simulink model "sim_all_2019b"  (R2019b)
settings: Solver=VariableStepAuto  StartTime=0.0  StopTime=2000  RelTol=1e-3
values from neighbouring files (symbols this model uses):
  nav_DT = 0.1    [navigation.m]
  nav_giro = 2    [navigation.m]
  nav_h0 = 0    [navigation.m]
  nav_lat0 = cornerC(1)    [navigation.m]
  nav_lon0 = cornerC(2)    [navigation.m]
  nav_plane_AB = coefficient_plane(nav_A,nav_B)    [navigation.m]
  nav_plane_BC = coefficient_plane(nav_B,nav_C)    [navigation.m]
  nav_plane_CD = coefficient_plane(nav_C,nav_D)    [navigation.m]
  nav_plane_DA = coefficient_plane(nav_D,nav_A)    [navigation.m]
undefined symbols (not defined in the file or in its folder): a1, a2, alpha1, alpha2, cornerA, cornerB, cornerC, cornerD, ctrl_clockwise, ctrl_int_bound_or, ctrl_int_bound_pos, ctrl_k_or, ctrl_k_pos, ctrl_Ki_vel, ctrl_Kp_v_pos, ctrl_Kp_vel, ctrl_TAM, ctrl_Ts, ctrl_va_uncontrolled, ctrl_vel_uncontrolled, D, dead_zone_limit, depth, DiscIntNeverNeededParam, distanceFromWall, initInspectedSide, initPoint, mod_A, mod_Cd_F, mod_Cd_M, mod_eta_init, mod_g, mod_h0, mod_Ixx, mod_Iyy, mod_Izz, mod_Kp_dot, mod_lat0, mod_lon0, mod_m, mod_Mq_dot, mod_ni_init, mod_Nr_dot, mod_p1, mod_p2, mod_p3, mod_p4, mod_p5, mod_p6, mod_R, mod_Rm, mod_t1, mod_t2, mod_t3, mod_t4, mod_t5, mod_t6, mod_W, mod_Xu_dot, mod_Yv_dot ... (+44)
libraries: simulink x8, cstblocks x6, simulink_extras x1
(part 1 of 6)
settings Model: PauseTimes=90  Creator=giorg  LastModifiedBy=Marco

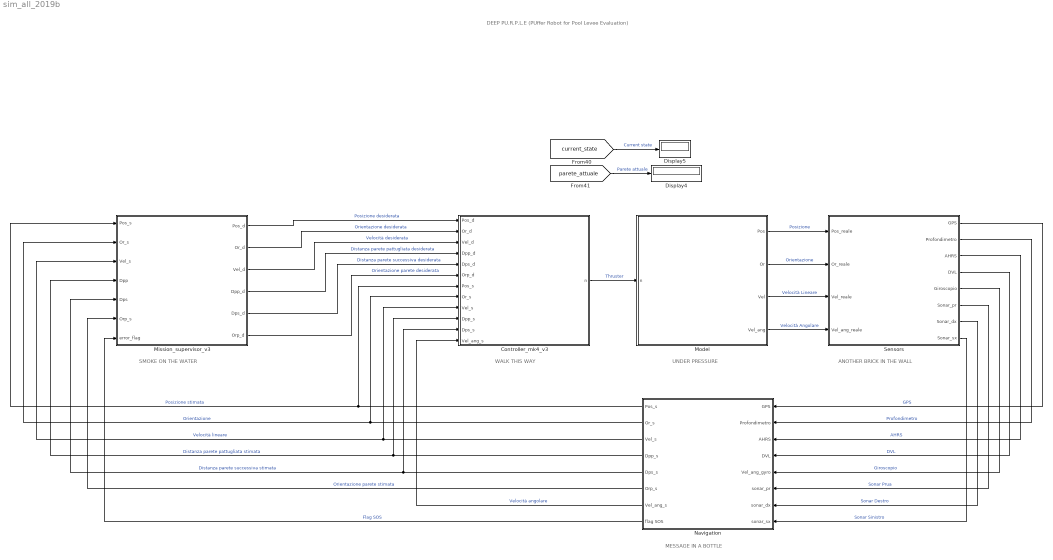
== system sim_all_2019b ==
  note: MESSAGE IN A BOTTLE
  note: ANOTHER BRICK IN THE WALL
  note: UNDER PRESSURE
  note: WALK THIS WAY
  note: SMOKE ON THE WATER
  note: DEEP PU.R.P.L.E
      | (PUffer Robot for Pool Levee Evaluation)
  Controller_mk4_v3 : Subsystem
  Display4 : Display
  Display5 : Display
  Mission_supervisor_v3 : Subsystem
  Model : Subsystem
  Navigation : Subsystem
  Sensors : Subsystem
  wires:
  [parete_attuale] -> Display4/1  "Parete attuale"
  [current_state] -> Display5/1  "Current state"
  Mission_supervisor_v3/1(Pos_d) -> Controller_mk4_v3/1(Pos_d)  "Posizione desiderata"
  Mission_supervisor_v3/2(Or_d) -> Controller_mk4_v3/2(Or_d)  "Orientazione desiderata"
  Mission_supervisor_v3/3(Vel_d) -> Controller_mk4_v3/3(Vel_d)  "Velocità desiderata"
  Mission_supervisor_v3/4(Dpp_d) -> Controller_mk4_v3/4(Dpp_d)  "Distanza parete pattugliata desiderata"
  Mission_supervisor_v3/5(Dps_d) -> Controller_mk4_v3/5(Dps_d)  "Distanza parete successiva desiderata"
  Mission_supervisor_v3/6(Orp_d) -> Controller_mk4_v3/6(Orp_d)  "Orientazione parete desiderata"
  Navigation/1(Pos_s) -> Controller_mk4_v3/7(Pos_s), Mission_supervisor_v3/1(Pos_s)  "Posizione stimata"
  Navigation/2(Or_s) -> Mission_supervisor_v3/2(Or_s), Controller_mk4_v3/8("Or_s ")  "Orientazione"
  Navigation/5(Dps_s) -> Mission_supervisor_v3/5(Dps), Controller_mk4_v3/11(Dps_s)  "Distanza parete successiva stimata"
  Navigation/4(Dpp_s) -> Mission_supervisor_v3/4(Dpp), Controller_mk4_v3/10(Dpp_s)  "Distanza parete pattugliata stimata"
  Navigation/3(Vel_s) -> Mission_supervisor_v3/3(Vel_s), Controller_mk4_v3/9(Vel_s)  "Velocità lineare"
  Controller_mk4_v3/1(n) -> Model/1(n)  "Thruster"
  Model/1(Pos) -> Sensors/1(Pos_reale)  "Posizione"
  Model/2(Or) -> Sensors/2(Or_reale)  "Orientazione"
  Model/4(Vel_ang) -> Sensors/4(Vel_ang_reale)  "Velocità Angolare"
  Navigation/7(Vel_ang_s) -> Controller_mk4_v3/12(Vel_ang_s)  "Velocità angolare"
  Model/3(Vel) -> Sensors/3(Vel_reale)  "Velocità Lineare"
  Sensors/1(GPS) -> Navigation/1(GPS)  "GPS"
  Sensors/5(Giroscopio) -> Navigation/5(Vel_ang_gyro)  "Giroscopio"
  Sensors/2(Profondimetro) -> Navigation/2(Profondimetro)  "Profondimetro"
  Navigation/6(Orp_s) -> Mission_supervisor_v3/6(Orp_s)  "Orientazione parete stimata"
  Navigation/8(flag SOS) -> Mission_supervisor_v3/7(error_flag)  "Flag SOS"
  Sensors/3(AHRS) -> Navigation/3(AHRS)  "AHRS"
  Sensors/6(Sonar_pr) -> Navigation/6(sonar_pr)  "Sonar Prua"
  Sensors/7(Sonar_dx) -> Navigation/7(sonar_dx)  "Sonar Destro"
  Sensors/8(Sonar_sx) -> Navigation/8(sonar_sx)  "Sonar Sinistro"
  Sensors/4(DVL) -> Navigation/4(DVL)  "DVL"

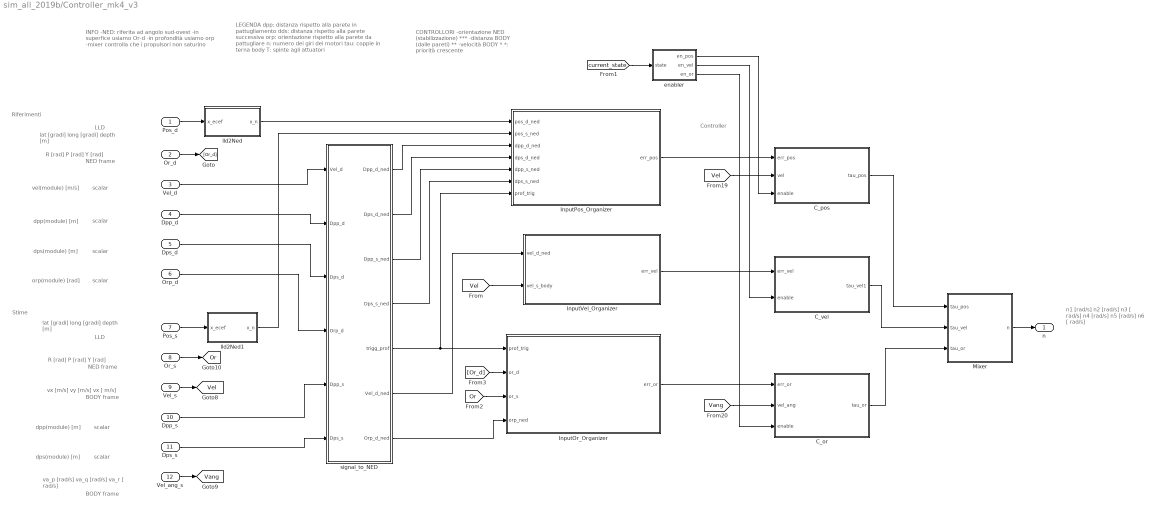
== system sim_all_2019b/Controller_mk4_v3 ==
  note: LEGENDA
      | dpp: distanza rispetto alla parete in pattugliamento
      | dds: distanza rispetto alla parete successiva
      | orp: orientazione rispetto alla parete da pattugliare
      | n: numero dei giri dei motori
      | tau: coppie in terna body
      | T: spinte agli attuatori
  note: CONTROLLORI
      | -orientazione NED (stabilizzazione) ***
      | -distanza BODY (dalle pareti) **
      | -velocità BODY *
      |
      | *: priorità crescente
  note: INFO
      | -NED: riferita ad angolo sud-ovest
      | -in superfice usiamo Or-d
      | -in profondità usiamo orp
      | -mixer controlla che i propulsori non saturino
  note: dpp(module) [m]
  note: LLD
  note: LLD
  note: orp(module) [rad]
  note: scalar
  note: va_p  [rad/s]
      | va_q  [rad/s]
      | va_r [ rad/s]
  note: lat  [gradi]
      | long  [gradi]
      | depth  [m]
  note: NED frame
  note: Controller
  note: dps(module) [m]
  note: BODY frame
  note: R  [rad]
      | P  [rad]
      | Y  [rad]
  note: scalar
  note: scalar
  note: R  [rad]
      | P  [rad]
      | Y  [rad]
  note: Stime
  note: Riferimenti
  note: n1  [rad/s]
      | n2  [rad/s]
      | n3 [ rad/s]
      | n4  [rad/s]
      | n5  [rad/s]
      | n6 [ rad/s]
  note: scalar
  note: vx  [m/s]
      | vy  [m/s]
      | vx [ m/s]
  note: scalar
  note: NED frame
  note: dpp(module) [m]
  note: scalar
  note: dps(module) [m]
  note: vel(module) [m/s]
  note: lat  [gradi]
      | long  [gradi]
      | depth  [m]
  note: BODY frame
  Pos_d : Inport  PortDimensions=[3 1]  SampleTime=ctrl_Ts
  Or_d : Inport  Port=2  PortDimensions=[3 1]  SampleTime=ctrl_Ts
  Vel_d : Inport  Port=3  PortDimensions=[1]  SampleTime=ctrl_Ts
  Dpp_d : Inport  Port=4  PortDimensions=[1]  SampleTime=ctrl_Ts
  Dps_d : Inport  Port=5  PortDimensions=[1]  SampleTime=ctrl_Ts
  Orp_d : Inport  Port=6  PortDimensions=[1]  SampleTime=ctrl_Ts
  Pos_s : Inport  Port=7  PortDimensions=[3 1]  SampleTime=ctrl_Ts
  "Or_s " : Inport  Port=8  PortDimensions=[3 1]  SampleTime=ctrl_Ts
  Vel_s : Inport  Port=9  PortDimensions=[3 1]  SampleTime=ctrl_Ts
  Dpp_s : Inport  Port=10  PortDimensions=[1]  SampleTime=ctrl_Ts
  Dps_s : Inport  Port=11  PortDimensions=[1]  SampleTime=ctrl_Ts
  Vel_ang_s : Inport  Port=12  PortDimensions=[3 1]  SampleTime=ctrl_Ts
  C_or : Subsystem
  C_pos : Subsystem
  C_vel : Subsystem
  InputOr_Organizer : Subsystem
  InputPos_Organizer : Subsystem
  InputVel_Organizer : Subsystem
  Mixer : Subsystem
  enabler : MATLAB Function  TreatAsAtomicUnit=on
  lld2Ned : MATLAB Function  TreatAsAtomicUnit=on
  lld2Ned1 : MATLAB Function  TreatAsAtomicUnit=on
  signal_to_NED : Subsystem
  n : Outport  PortDimensions=[6 1]
  tag scope: Or=global, Vang=global, Vel=global
  wires:
  lld2Ned/1(x_n) -> InputPos_Organizer/1(pos_d_ned)
  InputPos_Organizer/1(err_pos) -> C_pos/1(err_pos)
  enabler/3(en_or) -> C_or/3(enable)
  Pos_s/1 -> lld2Ned1/1(x_ecef)
  [Vel] -> C_pos/2(vel)
  Pos_d/1 -> lld2Ned/1(x_ecef)
  [current_state] -> enabler/1(state)
  [Vang] -> C_or/2(vel_ang)
  C_vel/1(tau_vel1) -> Mixer/2(tau_vel)
  C_or/1(tau_or) -> Mixer/3(tau_or)
  C_pos/1(tau_pos) -> Mixer/1(tau_pos)
  enabler/1(en_pos) -> C_pos/3(enable)
  InputOr_Organizer/1(err_or) -> C_or/1(err_or)
  InputVel_Organizer/1(err_vel) -> C_vel/1(err_vel)
  lld2Ned1/1(x_n) -> InputPos_Organizer/2(pos_s_ned)
  Vel_ang_s/1 -> [Vang]
  signal_to_NED/5(trigg_prof) -> InputPos_Organizer/7(prof_trig), InputOr_Organizer/1(prof_trig)
  signal_to_NED/7(Orp_d_ned) -> InputOr_Organizer/4(orp_ned)
  Vel_d/1 -> signal_to_NED/1(Vel_d)
  Dpp_d/1 -> signal_to_NED/2(Dpp_d)
  Dps_d/1 -> signal_to_NED/3(Dps_d)
  Orp_d/1 -> signal_to_NED/4(Orp_d)
  Dpp_s/1 -> signal_to_NED/5(Dpp_s)
  Dps_s/1 -> signal_to_NED/6(Dps_s)
  signal_to_NED/1(Dpp_d_ned) -> InputPos_Organizer/3(dpp_d_ned)
  signal_to_NED/2(Dps_d_ned) -> InputPos_Organizer/4(dps_d_ned)
  signal_to_NED/3(Dpp_s_ned) -> InputPos_Organizer/5(dpp_s_ned)
  signal_to_NED/4(Dps_s_ned) -> InputPos_Organizer/6(dps_s_ned)
  signal_to_NED/6(Vel_d_ned) -> InputVel_Organizer/1(vel_d_ned)
  "Or_s "/1 -> [Or]
  Vel_s/1 -> [Vel]
  [Vel] -> InputVel_Organizer/2(vel_s_body)
  [Or] -> InputOr_Organizer/3(or_s)
  Or_d/1 -> [Or_d]
  [Or_d] -> InputOr_Organizer/2(or_d)
  enabler/2(en_vel) -> C_vel/2(enable)
  Mixer/1(n) -> n/1

== system sim_all_2019b/Mission_supervisor_v3 ==
  note: Orp [deg]
  note: Vel [m/s]
  note: Dpp [m]
  note: R  [rad]
      | P  [rad]
      | Y  [rad]
  note: ECEF
      | ECEF
      | NED
  note: Roll  [rad]
      | Pitch  [rad]
      | Yaw  [rad]
  note: vx  [m/s]
      | vy  [m/s]
      | vx  [m/s]
  note: BODY frame
  note: ECEF
      | ECEF
      | NED
  note: lat  [gradi]
      | long  [gradi]
      | depth  [m]
  note: Dps [m]
  note: Dpp [m]
  note: Dpp: distanza dalla parete pattugliata
      | Dps: Distanza dalla parete successiva
      | Orp: orientazione rispetto alla parete pattugliata
      | Or_d: orientazione in superficie
  note: Dps [m]
  note: Orp [rad]
  note: lat  [gradi]
      | long  [gradi]
      | depth   [m]
  Pos_s : Inport  PortDimensions=[3 1]
  Or_s : Inport  Port=2  PortDimensions=[3 1]
  Vel_s : Inport  Port=3  PortDimensions=[3 1]
  Dpp : Inport  Port=4  PortDimensions=1
  Dps : Inport  Port=5  PortDimensions=1
  Orp_s : Inport  Port=6  PortDimensions=1
  error_flag : Inport  Port=7  PortDimensions=1
  Display4 : Display
  Display5 : Display
  Mission_Supervisor : Subsystem
  Pos_d : Outport  PortDimensions=[3 1]
  Or_d : Outport  Port=2  PortDimensions=[3 1]
  Vel_d : Outport  Port=3  PortDimensions=1
  Dpp_d : Outport  Port=4  PortDimensions=1
  Dps_d : Outport  Port=5  PortDimensions=1
  Orp_d : Outport  Port=6  PortDimensions=1
  wires:
  [current_state] -> Display5/1
  Mission_Supervisor/5(Dps_d) -> Dps_d/1
  Mission_Supervisor/4(Dpp_d) -> Dpp_d/1
  Dps/1 -> Mission_Supervisor/5(Dps)
  Mission_Supervisor/3(Vel_d) -> Vel_d/1
  error_flag/1 -> Mission_Supervisor/7(error_flag)
  Pos_s/1 -> Mission_Supervisor/1(Pos_S)
  Vel_s/1 -> Mission_Supervisor/3(Vel_S)
  Mission_Supervisor/1(Pos_d) -> Pos_d/1
  Mission_Supervisor/6(Orp_d) -> Orp_d/1
  Dpp/1 -> Mission_Supervisor/4(Dpp)
  [parete_attuale] -> Display4/1
  Orp_s/1 -> Mission_Supervisor/6(Orp_s)
  Mission_Supervisor/2(Or_d) -> Or_d/1
  Or_s/1 -> Mission_Supervisor/2(Or_S)

== system sim_all_2019b/Model ==
  note: Body frame
      | u [m/s]
      | v [m/s]
      | w [m/s]
  note: Body frame
      | p [rad/s]
      | q [rad/s]
      | r [rad/s]
  note: ECEF frame
      | lat [deg]
      | long [deg]
      | depth [m]
  note: NED frame
      | R [rad]
      | P [rad]
      | Y [rad]
  n : Inport  PortDimensions=[6 1]
  Demux : Demux  Outputs=6
  Demux1 : Demux  Outputs=2
  Demux2 : Demux  Outputs=2
  Orientation in Deg : Scope  Commented=on
  Position in ECEF : Scope  Commented=on
  Vehicle Model : Subsystem
  from NED to ECEF : MATLAB Function  TreatAsAtomicUnit=on
  from Rad to Deg : MATLAB Function  TreatAsAtomicUnit=on
  Pos : Outport  PortDimensions=[3 1]
  Or : Outport  Port=2  PortDimensions=[3 1]
  Vel : Outport  Port=3  PortDimensions=[3 1]
  Vel_ang : Outport  Port=4  PortDimensions=[3 1]
  wires:
  n/1 -> Demux/1
  from Rad to Deg/1(eta2_deg) -> Orientation in Deg/1  "eta2_deg"
  Vehicle Model/2(ni) -> Demux1/1
  Demux/3 -> Vehicle Model/3(In3)
  Demux/4 -> Vehicle Model/4(In4)
  from NED to ECEF/1(eta1_ECEF) -> Position in ECEF/1, Pos/1  "eta1_ECEF"
  Vehicle Model/1(eta) -> Demux2/1
  Demux/6 -> Vehicle Model/6(In6)
  Demux/1 -> Vehicle Model/1(In1)
  Demux/5 -> Vehicle Model/5(In5)
  Demux2/1 -> from NED to ECEF/1(eta1)  "Posizione Reale NED"
  Demux1/2 -> Vel_ang/1  "ni2"
  Demux1/1 -> Vel/1  "ni1"
  Demux2/2 -> Or/1, from Rad to Deg/1(eta2)  "eta2"
  Demux/2 -> Vehicle Model/2(In2)

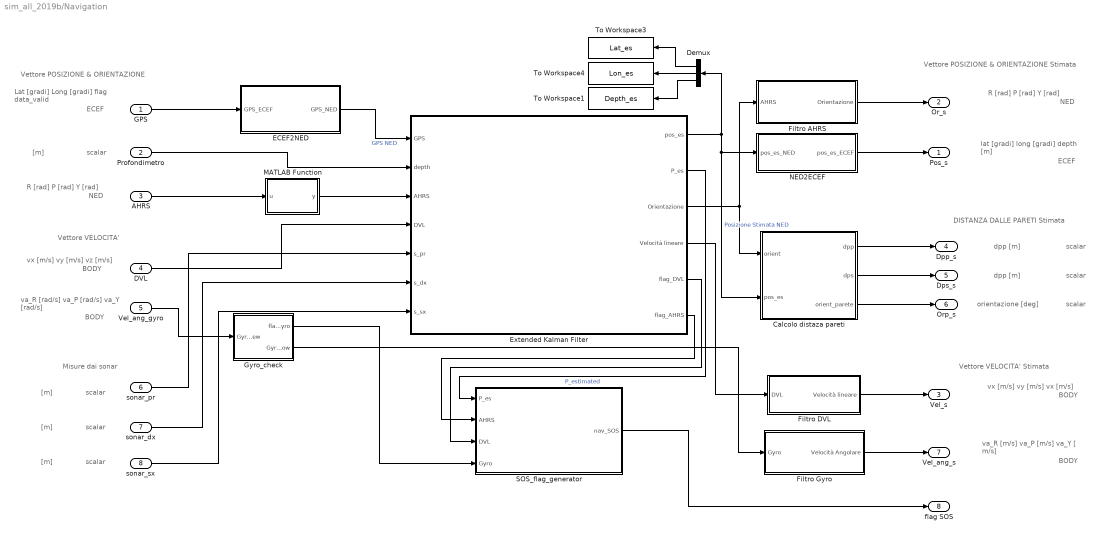
== system sim_all_2019b/Navigation ==
  note: Vettore POSIZIONE & ORIENTAZIONE
  note: vx  [m/s]
      | vy  [m/s]
      | vx  [m/s]
  note: R [rad]
      | P [rad]
      | Y [rad]
  note: vx  [m/s]
      | vy  [m/s]
      | vz  [m/s]
  note: scalar
  note: dpp [m]
  note: [m]
  note: [m]
  note: NED
  note: ECEF
  note: lat  [gradi]
      | long  [gradi]
      | depth   [m]
  note: va_R [rad/s]
      | va_P [rad/s]
      | va_Y [rad/s]
  note: NED
  note: va_R  [m/s]
      | va_P  [m/s]
      | va_Y [ m/s]
  note: BODY
  note: [m]
  note: BODY
  note: Lat  [gradi]
      | Long  [gradi]
      | flag data_valid
  note: ECEF
  note: R  [rad]
      | P  [rad]
      | Y  [rad]
  note: scalar
  note: BODY
  note: scalar
  note: scalar
  note: scalar
  note: scalar
  note: BODY
  note: [m]
  note: Vettore POSIZIONE & ORIENTAZIONE Stimata
  note: Vettore VELOCITA'
  note: DISTANZA DALLE PARETI Stimata
  note: Vettore VELOCITA' Stimata
  note: Misure dai sonar
  note: dpp [m]
  note: orientazione [deg]
  note: scalar
  GPS : Inport  PortDimensions=[3 1]
  Profondimetro : Inport  Port=2  PortDimensions=1
  AHRS : Inport  Port=3  PortDimensions=[3 1]
  DVL : Inport  Port=4  PortDimensions=[3 1]
  Vel_ang_gyro : Inport  Port=5  PortDimensions=[3 1]
  sonar_pr : Inport  Port=6  PortDimensions=1
  sonar_dx : Inport  Port=7  PortDimensions=1
  sonar_sx : Inport  Port=8  PortDimensions=1
  Calcolo distaza pareti : Subsystem
  Demux : Demux  Outputs=3
  ECEF2NED : MATLAB Function  TreatAsAtomicUnit=on
  Extended Kalman Filter : Subsystem  TreatAsAtomicUnit=on
  Filtro AHRS : Subsystem
  Filtro DVL : Subsystem
  Filtro Gyro : Subsystem
  Gyro_check : Subsystem
  MATLAB Function : MATLAB Function  TreatAsAtomicUnit=on
  NED2ECEF : MATLAB Function  TreatAsAtomicUnit=on
  SOS_flag_generator : Subsystem
  To Workspace1 : ToWorkspace  VariableName=Depth_es  SaveFormat=Timeseries  SampleTime=-1
      settings: Decimation=10
  To Workspace3 : ToWorkspace  VariableName=Lat_es  SaveFormat=Timeseries  SampleTime=-1
      settings: Decimation=10
  To Workspace4 : ToWorkspace  VariableName=Lon_es  SaveFormat=Timeseries  SampleTime=-1
      settings: Decimation=10
  Pos_s : Outport  PortDimensions=[3 1]
  Or_s : Outport  Port=2  PortDimensions=[3 1]
  Vel_s : Outport  Port=3  PortDimensions=[3 1]
  Dpp_s : Outport  Port=4  PortDimensions=1
  Dps_s : Outport  Port=5  PortDimensions=1
  Orp_s : Outport  Port=6  PortDimensions=1
  Vel_ang_s : Outport  Port=7  PortDimensions=[3 1]
  flag SOS : Outport  Port=8  PortDimensions=1
  wires:
  Profondimetro/1 -> Extended Kalman Filter/2(depth)
  sonar_pr/1 -> Extended Kalman Filter/5(s_pr)
  sonar_dx/1 -> Extended Kalman Filter/6(s_dx)
  sonar_sx/1 -> Extended Kalman Filter/7(s_sx)
  Extended Kalman Filter/1(pos_es) -> Calcolo distaza pareti/2(pos_es), NED2ECEF/1(pos_es_NED), Demux/1  "Posizione Stimata NED"
  Calcolo distaza pareti/1(dpp) -> Dpp_s/1
  Calcolo distaza pareti/2(dps) -> Dps_s/1
  NED2ECEF/1(pos_es_ECEF) -> Pos_s/1
  GPS/1 -> ECEF2NED/1(GPS_ECEF)
  ECEF2NED/1(GPS_NED) -> Extended Kalman Filter/1(GPS)  "GPS NED"
  Calcolo distaza pareti/3(orient_parete) -> Orp_s/1
  Extended Kalman Filter/2(P_es) -> SOS_flag_generator/1(P_es)  "P_estimated"
  AHRS/1 -> MATLAB Function/1(u)
  Filtro DVL/1(Velocità lineare) -> Vel_s/1
  Filtro AHRS/1(Orientazione) -> Or_s/1
  Filtro Gyro/1(Velocità Angolare) -> Vel_ang_s/1
  MATLAB Function/1(y) -> Extended Kalman Filter/3(AHRS)
  Extended Kalman Filter/3(Orientazione) -> Calcolo distaza pareti/1(orient), Filtro AHRS/1(AHRS)
  Vel_ang_gyro/1 -> Gyro_check/1(Gyro_new)
  Gyro_check/2(Gyro_now) -> Filtro Gyro/1(Gyro)
  Extended Kalman Filter/5(flag_DVL) -> SOS_flag_generator/3(DVL)
  Extended Kalman Filter/6(flag_AHRS) -> SOS_flag_generator/2(AHRS)
  Gyro_check/1(flag_Gyro) -> SOS_flag_generator/4(Gyro)
  SOS_flag_generator/1(nav_SOS) -> flag SOS/1
  DVL/1 -> Extended Kalman Filter/4(DVL)
  Extended Kalman Filter/4(Velocità lineare) -> Filtro DVL/1(DVL)
  Demux/2 -> To Workspace4/1
  Demux/1 -> To Workspace3/1
  Demux/3 -> To Workspace1/1

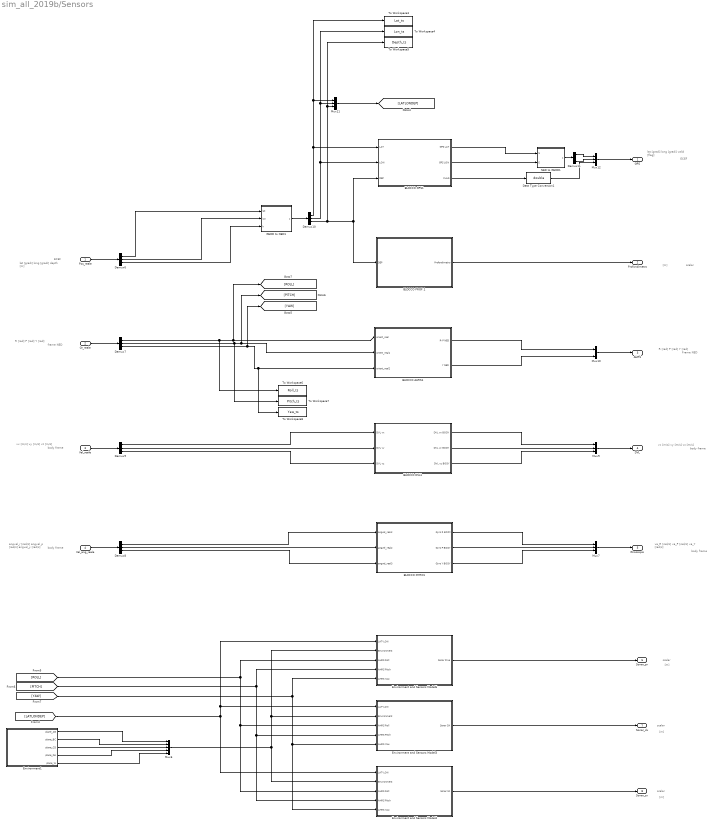
== system sim_all_2019b/Sensors ==
  note: body frame
  note: body frame
  note: ECEF
  note: scalar
  note: [m]
  note: [m]
  note: R  [rad]
      | P  [rad]
      | Y  [rad]
  note: ECEF
  note: va_R [rad/s]
      | va_P [rad/s]
      | va_Y [rad/s]
  note: Frame NED
  note: lat  [gradi]
      | long  [gradi]
      | valid [flag]
  note: body frame
  note: [m]
  note: angvel_r  [rad/s]
      | angvel_p  [rad/s]
      | angvel_y  [rad/s]
  note: vx  [m/s]
      | vy  [m/s]
      | vz  [m/s]
  note: frame NED
  note: lat  [gradi]
      | long  [gradi]
      | depth  [m]
  note: scalar
  note: vx  [m/s]
      | vy  [m/s]
      | vz  [m/s]
  note: scalar
  note: body frame
  note: [m]
  note: scalar
  note: R  [rad]
      | P  [rad]
      | Y  [rad]
  Pos_reale : Inport  PortDimensions=[3 1]
  Or_reale : Inport  Port=2  PortDimensions=[3 1]
  Vel_reale : Inport  Port=3  PortDimensions=[3 1]
  Vel_ang_reale : Inport  Port=4  PortDimensions=[3 1]
  BLOCCO AHRS1 : Subsystem
  BLOCCO DVL1 : Subsystem
  BLOCCO GPS1 : Subsystem
  BLOCCO GYRO1 : Subsystem
  BLOCCO PROF.1 : Subsystem
  Data Type Conversion1 : DataTypeConversion  OutDataTypeStr=double
  Demux{6..10} (5 alike) : Demux  Outputs=3
  Demux11 : Demux  Outputs=2
  Environment and Sensors Model3 : Subsystem
  Environment and Sensors Model4 : Subsystem
  Environment and Sensors Model6 : Subsystem
  Environment1 : MATLAB Function  TreatAsAtomicUnit=on
  GEOD to NED1 : MATLAB Function  TreatAsAtomicUnit=on
  Mux10 : Mux  Inputs=2
  Mux{7,9,11..12} (4 alike) : Mux  Inputs=3
  Mux6 : Mux  Inputs=5
  NED to GEOD1 : MATLAB Function  TreatAsAtomicUnit=on
  To Workspace3 : ToWorkspace  VariableName=Lat_ts  SaveFormat=Timeseries  SampleTime=-1
      settings: Decimation=10
  To Workspace4 : ToWorkspace  VariableName=Lon_ts  SaveFormat=Timeseries  SampleTime=-1
      settings: Decimation=10
  To Workspace5 : ToWorkspace  VariableName=Depth_ts  SaveFormat=Timeseries  SampleTime=-1
      settings: Decimation=10
  To Workspace6 : ToWorkspace  VariableName=Roll_ts  SaveFormat=Timeseries  SampleTime=-1
      settings: Decimation=10
  To Workspace7 : ToWorkspace  VariableName=Pitch_ts  SaveFormat=Timeseries  SampleTime=-1
      settings: Decimation=10
  To Workspace8 : ToWorkspace  VariableName=Yaw_ts  SaveFormat=Timeseries  SampleTime=-1
      settings: Decimation=10
  GPS : Outport  PortDimensions=[3 1]
  Profondimetro : Outport  Port=2  PortDimensions=1
  AHRS : Outport  Port=3  PortDimensions=[3 1]
  DVL : Outport  Port=4  PortDimensions=[3 1]
  Giroscopio : Outport  Port=5  PortDimensions=[3 1]
  Sonar_pr : Outport  Port=6  PortDimensions=1
  Sonar_dx : Outport  Port=7  PortDimensions=1
  Sonar_sx : Outport  Port=8  PortDimensions=1
  wires:
  Environment1/5(plane_W) -> Mux6/5
  Demux10/2 -> BLOCCO GPS1/2("LON "), To Workspace4/1, Mux11/2
  Demux10/1 -> To Workspace3/1, Mux11/1, BLOCCO GPS1/1("LAT ")
  BLOCCO DVL1/2(DVL vy BODY) -> Mux9/2
  Environment and Sensors Model6/1(Sonar Prua) -> Sonar_pr/1
  BLOCCO AHRS1/1(R-P NED) -> Mux10/1
  BLOCCO GYRO1/3(Gyro Y BODY) -> Mux7/3
  Demux9/3 -> BLOCCO DVL1/3(DVL vz)
  Demux10/3 -> BLOCCO GPS1/3(DEP), BLOCCO PROF.1/1(DEP), To Workspace5/1, Mux11/3
  Demux9/2 -> BLOCCO DVL1/2(DVL vy)
  BLOCCO GYRO1/1(Gyro R BODY) -> Mux7/1
  BLOCCO DVL1/1(DVL vx BODY) -> Mux9/1
  BLOCCO AHRS1/2(Y NED) -> Mux10/2
  Environment1/2(plane_BC) -> Mux6/2
  Pos_reale/1 -> Demux6/1
  BLOCCO GYRO1/2(Gyro P BODY) -> Mux7/2
  Vel_ang_reale/1 -> Demux8/1
  Environment1/3(plane_CD) -> Mux6/3
  [YAW] -> Environment and Sensors Model3/5(AHRS Yaw), Environment and Sensors Model4/5(AHRS Yaw), Environment and Sensors Model6/5(AHRS Yaw)
  Mux6/1 -> Environment and Sensors Model3/2(Environment), Environment and Sensors Model6/2(Environment), Environment and Sensors Model4/2(Environment)
  Vel_reale/1 -> Demux9/1
  Demux6/2 -> GEOD to NED1/2(lon)
  Data Type Conversion1/1 -> Mux12/3
  Demux11/2 -> Mux12/2
  Or_reale/1 -> Demux7/1
  Demux8/3 -> BLOCCO GYRO1/3(angvel_real3)
  BLOCCO DVL1/3(DVL vz BODY) -> Mux9/3
  Mux10/1 -> AHRS/1
  Demux7/1 -> To Workspace6/1, BLOCCO AHRS1/1(orient_real), [ROLL]
  Demux7/2 -> To Workspace7/1, BLOCCO AHRS1/2(orient_real1), [PITCH]
  Demux6/1 -> GEOD to NED1/1(lat)
  [PITCH] -> Environment and Sensors Model6/4(AHRS Pitch), Environment and Sensors Model3/4(AHRS Pitch), Environment and Sensors Model4/4(AHRS Pitch)
  Demux8/1 -> BLOCCO GYRO1/1(angvel_rea1l)
  Demux7/3 -> To Workspace8/1, BLOCCO AHRS1/3(orient_real2), [YAW]
  Demux6/3 -> GEOD to NED1/3(h)
  Mux11/1 -> [LATLONDEP]
  Mux9/1 -> DVL/1
  Environment and Sensors Model4/1(Sonar SX) -> Sonar_sx/1
  Mux7/1 -> Giroscopio/1
  BLOCCO GPS1/3(FLAG) -> Data Type Conversion1/1
  BLOCCO PROF.1/1(Profondimetro) -> Profondimetro/1
  [ROLL] -> Environment and Sensors Model6/3(AHRS Roll), Environment and Sensors Model3/3(AHRS Roll), Environment and Sensors Model4/3(AHRS Roll)
  BLOCCO GPS1/2("GPS LON ") -> NED to GEOD1/2(E)
  GEOD to NED1/1(z) -> Demux10/1
  Demux8/2 -> BLOCCO GYRO1/2(angvel_real2)
  Demux9/1 -> BLOCCO DVL1/1("DVL vx ")
  BLOCCO GPS1/1("GPS LAT ") -> NED to GEOD1/1(N)
  [LATLONDEP] -> Environment and Sensors Model3/1(LAT-LON), Environment and Sensors Model6/1(LAT-LON), Environment and Sensors Model4/1(LAT-LON)
  NED to GEOD1/1(z) -> Demux11/1
  Demux11/1 -> Mux12/1
  Environment1/1(plane_AB) -> Mux6/1
  Environment and Sensors Model3/1(Sonar DX) -> Sonar_dx/1
  Environment1/4(plane_DA) -> Mux6/4
  Mux12/1 -> GPS/1

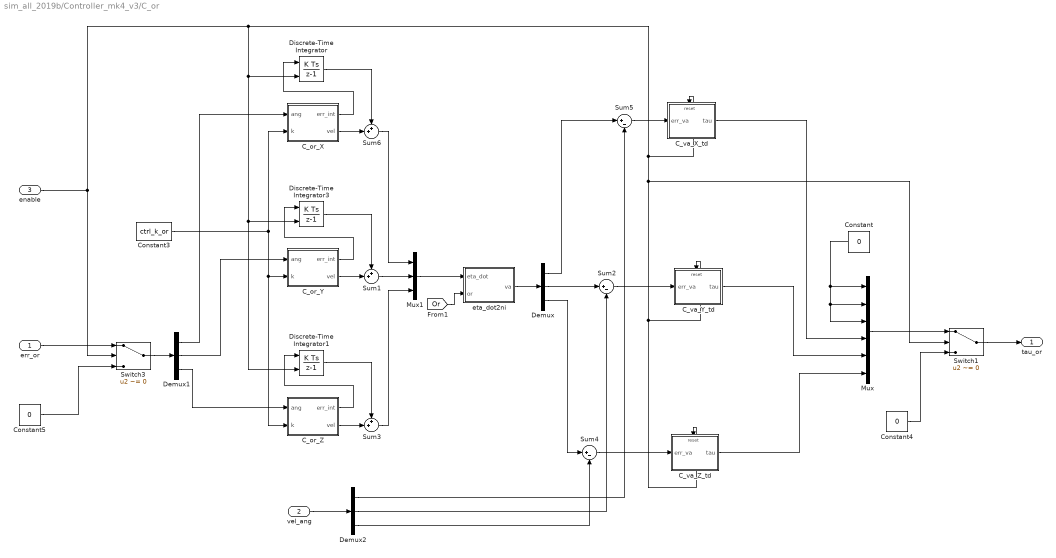
== system sim_all_2019b/Controller_mk4_v3/C_or ==
  err_or : Inport
  vel_ang : Inport  Port=2
  enable : Inport  Port=3
  C_or_X : MATLAB Function  TreatAsAtomicUnit=on  SystemSampleTime=ctrl_Ts
  C_or_Y : MATLAB Function  TreatAsAtomicUnit=on  SystemSampleTime=ctrl_Ts
  C_or_Z : MATLAB Function  TreatAsAtomicUnit=on  SystemSampleTime=ctrl_Ts
  C_va_X_td : Subsystem  TreatAsAtomicUnit=on
  C_va_Y_td : Subsystem  TreatAsAtomicUnit=on
  C_va_Z_td : Subsystem  TreatAsAtomicUnit=on
  Constant : Constant  Value=0
  Constant3 : Constant  Value=ctrl_k_or
  Constant4 : Constant  Value=0
  Constant5 : Constant  Value=0
  Demux : Demux  Outputs=3
  Demux1 : Demux  Outputs=3
  Demux2 : Demux  Outputs=3
  Discrete-Time Integrator : DiscreteIntegrator  gainval=ctrl_Ki_or  ExternalReset=rising  SampleTime=ctrl_Ts  ICPrevOutput=DiscIntNeverNeededParam  ICPrevScaledInput=DiscIntNeverNeededParam
  Discrete-Time Integrator1 : DiscreteIntegrator  gainval=ctrl_Ki_or  ExternalReset=rising  SampleTime=ctrl_Ts  ICPrevOutput=DiscIntNeverNeededParam  ICPrevScaledInput=DiscIntNeverNeededParam
  Discrete-Time Integrator3 : DiscreteIntegrator  gainval=ctrl_Ki_or  ExternalReset=rising  SampleTime=ctrl_Ts  ICPrevOutput=DiscIntNeverNeededParam  ICPrevScaledInput=DiscIntNeverNeededParam
  Mux : Mux  Inputs=6
  Mux1 : Mux  Inputs=3
  Sum1 : Sum  Inputs=++|
  Sum2 : Sum  Inputs=|+-
  Sum3 : Sum  Inputs=++|
  Sum4 : Sum  Inputs=|+-
  Sum5 : Sum  Inputs=|+-
  Sum6 : Sum  Inputs=++|
  Switch1 : Switch  Criteria=u2 ~= 0  Threshold=0.5
  Switch3 : Switch  Criteria=u2 ~= 0  Threshold=0.5
  eta_dot2ni : MATLAB Function  TreatAsAtomicUnit=on  SystemSampleTime=ctrl_Ts
  tau_or : Outport  VectorParamsAs1DForOutWhenUnconnected=off
  wires:
  Sum5/1 -> C_va_X_td/1(err_va)
  Demux2/1 -> Sum5/2
  Sum2/1 -> C_va_Y_td/1(err_va)
  Constant/1 -> Mux/1, Mux/3, Mux/2
  C_va_X_td/1(tau) -> Mux/4
  C_va_Y_td/1(tau) -> Mux/5
  Constant3/1 -> C_or_Z/2(k), C_or_Y/2(k), C_or_X/2(k)
  Sum4/1 -> C_va_Z_td/1(err_va)
  Demux2/2 -> Sum2/2
  Demux2/3 -> Sum4/2
  vel_ang/1 -> Demux2/1
  Constant4/1 -> Switch1/3
  Mux/1 -> Switch1/1
  Switch1/1 -> tau_or/1
  Constant5/1 -> Switch3/3
  Switch3/1 -> Demux1/1
  err_or/1 -> Switch3/1
  Demux1/3 -> C_or_Z/1(ang)
  Demux1/2 -> C_or_Y/1(ang)
  Demux1/1 -> C_or_X/1(ang)
  C_va_Z_td/1(tau) -> Mux/6
  [Or] -> eta_dot2ni/2(or)
  eta_dot2ni/1(va) -> Demux/1
  Demux/2 -> Sum2/1
  Mux1/1 -> eta_dot2ni/1(eta_dot)
  Demux/1 -> Sum5/1
  Demux/3 -> Sum4/1
  Sum6/1 -> Mux1/1
  Sum1/1 -> Mux1/2
  Sum3/1 -> Mux1/3
  enable/1 -> Switch3/2, Discrete-Time Integrator1/2, Discrete-Time Integrator3/2, Discrete-Time Integrator/2, Switch1/2, C_va_Z_td/Reset, C_va_Y_td/Reset, C_va_X_td/Reset
  C_or_Z/1(err_int) -> Discrete-Time Integrator1/1
  C_or_Y/1(err_int) -> Discrete-Time Integrator3/1
  C_or_X/1(err_int) -> Discrete-Time Integrator/1
  C_or_X/2(vel) -> Sum6/2
  C_or_Z/2(vel) -> Sum3/2
  Discrete-Time Integrator3/1 -> Sum1/1
  Discrete-Time Integrator/1 -> Sum6/1
  Discrete-Time Integrator1/1 -> Sum3/1
  C_or_Y/2(vel) -> Sum1/2

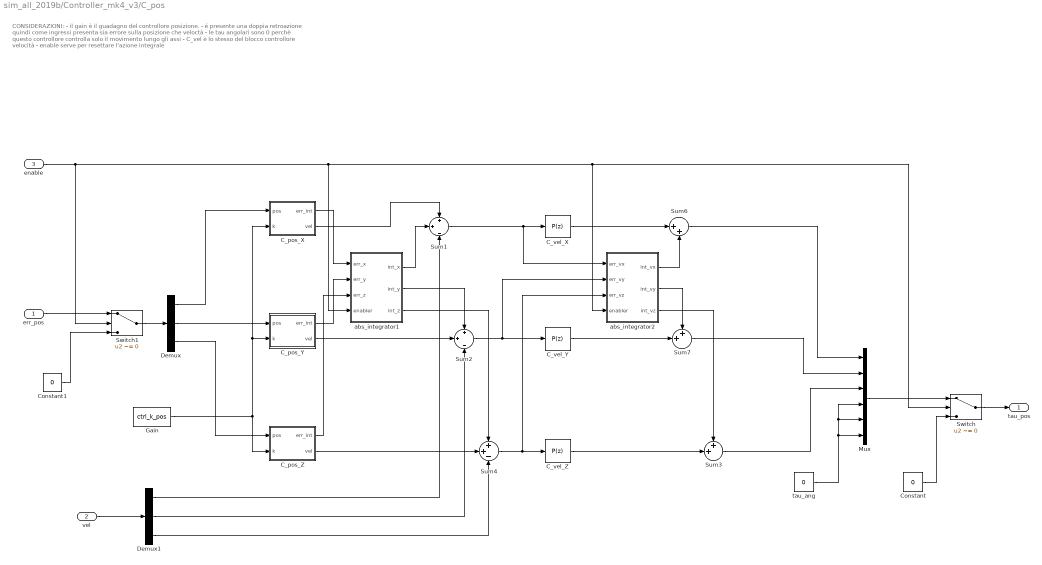
== system sim_all_2019b/Controller_mk4_v3/C_pos ==
  note: CONSIDERAZIONI:
      | - il gain è il guadagno del controllore posizione.
      | - é presente una doppia retroazione quindi come ingressi presenta sia errore sulla posizione che veloctà
      | - le tau angolari sono 0 perchè questo controllore controlla solo il movimento lungo gli assi
      | - C_vel è lo stesso del blocco controllore velocità
      | - enable serve per resettare l'azione integrale
  err_pos : Inport
  vel : Inport  Port=2
  enable : Inport  Port=3
  C_pos_X : MATLAB Function  TreatAsAtomicUnit=on
  C_pos_Y : MATLAB Function  TreatAsAtomicUnit=on
  C_pos_Z : MATLAB Function  TreatAsAtomicUnit=on
  C_vel_X : simulink/Continuous/PID Controller  Controller=P  Form=Parallel  TimeDomain=Discrete-time  SampleTime=ctrl_Ts  IntegratorMethod=Forward Euler  FilterMethod=Forward Euler  ControllerParametersSource=internal  P=ctrl_Kp_v_pos  I=ctrl_Ki_vel  D=0  UseFilter=on  N=100  TunerSelectOption=Transfer Function Based (PID Tuner App)  InitialConditionSource=internal  InitialConditionForIntegrator=0  InitialConditionForFilter=0  DifferentiatorICPrevScaledInput=0  ExternalReset=rising  TrackingMode=off  Kt=1  LimitOutput=off  UpperSaturationLimit=inf  LowerSaturationLimit=-inf  LinearizeAsGain=on  AntiWindupMode=none  Kb=1  POutMin=[]  POutMax=[]  IOutMin=[]  IOutMax=[]  DOutMin=[]  DOutMax=[]  NOutMin=[]  NOutMax=[]  SumOutMin=[]  SumOutMax=[]  SaturationOutMin=[]  SaturationOutMax=[]  PParamMin=[]  PParamMax=[]  IParamMin=[]  IParamMax=[]  DParamMin=[]  DParamMax=[]  NParamMin=[]  NParamMax=[]  KbParamMin=[]  KbParamMax=[]  KtParamMin=[]  KtParamMax=[]  KbOutMin=[]  KbOutMax=[]  KtOutMin=[]  KtOutMax=[]  IntegratorOutMin=[]  IntegratorOutMax=[]  FilterOutMin=[]  FilterOutMax=[]  SumI1OutMin=[]  SumI1OutMax=[]  SumI2OutMin=[]  SumI2OutMax=[]  SumI3OutMin=[]  SumI3OutMax=[]  SumI4OutMin=[]  SumI4OutMax=[]  SumDOutMin=[]  SumDOutMax=[]  DifferentiatorOutMin=[]  DifferentiatorOutMax=[]  FilterDiffOutCoefMin=[]  FilterDiffOutCoefMax=[]  ReciprocalOutMin=[]  ReciprocalOutMax=[]  SumDenOutMin=[]  SumDenOutMax=[]  SumNumOutMin=[]  SumNumOutMax=[]  DivideOutMin=[]  DivideOutMax=[]  IntegratorContinuousStateAttributes=''  IntegratorStateMustResolveToSignalObject=off  IntegratorRTWStateStorageClass=Auto  FilterContinuousStateAttributes=''  FilterStateMustResolveToSignalObject=off  FilterRTWStateStorageClass=Auto  ParallelPVariant=InternalParameters  IdealPVariant=Disabled  IVariant=Disabled  DVariant=Disabled  IntegratorVariant=Disabled  SatVariant=Disabled  AWVariant=Disabled  PCopyVariant=Disabled  TRVariant=Disabled  FdbkBlocksVariant=Forward  IdealPFdbkVariant=Disabled  SatFdbkVariant=Disabled  DerivativeFilterVariant=Disabled  NVariant=Disabled  NCopyVariant=Disabled_SignalSpec  FilterICVariant=Disabled  IntegratorICVariant=Disabled  ExternalResetVariant=Disabled  TRSumVariant=Passthrough  SumFdbkVariant=Disabled  SumVariant=Passthrough_P
  C_vel_Y : simulink/Continuous/PID Controller  Controller=P  Form=Parallel  TimeDomain=Discrete-time  SampleTime=ctrl_Ts  IntegratorMethod=Forward Euler  FilterMethod=Forward Euler  ControllerParametersSource=internal  P=ctrl_Kp_v_pos  I=ctrl_Ki_vel  D=0  UseFilter=on  N=100  TunerSelectOption=Transfer Function Based (PID Tuner App)  InitialConditionSource=internal  InitialConditionForIntegrator=0  InitialConditionForFilter=0  DifferentiatorICPrevScaledInput=0  ExternalReset=rising  TrackingMode=off  Kt=1  LimitOutput=off  UpperSaturationLimit=inf  LowerSaturationLimit=-inf  LinearizeAsGain=on  AntiWindupMode=none  Kb=1  POutMin=[]  POutMax=[]  IOutMin=[]  IOutMax=[]  DOutMin=[]  DOutMax=[]  NOutMin=[]  NOutMax=[]  SumOutMin=[]  SumOutMax=[]  SaturationOutMin=[]  SaturationOutMax=[]  PParamMin=[]  PParamMax=[]  IParamMin=[]  IParamMax=[]  DParamMin=[]  DParamMax=[]  NParamMin=[]  NParamMax=[]  KbParamMin=[]  KbParamMax=[]  KtParamMin=[]  KtParamMax=[]  KbOutMin=[]  KbOutMax=[]  KtOutMin=[]  KtOutMax=[]  IntegratorOutMin=[]  IntegratorOutMax=[]  FilterOutMin=[]  FilterOutMax=[]  SumI1OutMin=[]  SumI1OutMax=[]  SumI2OutMin=[]  SumI2OutMax=[]  SumI3OutMin=[]  SumI3OutMax=[]  SumI4OutMin=[]  SumI4OutMax=[]  SumDOutMin=[]  SumDOutMax=[]  DifferentiatorOutMin=[]  DifferentiatorOutMax=[]  FilterDiffOutCoefMin=[]  FilterDiffOutCoefMax=[]  ReciprocalOutMin=[]  ReciprocalOutMax=[]  SumDenOutMin=[]  SumDenOutMax=[]  SumNumOutMin=[]  SumNumOutMax=[]  DivideOutMin=[]  DivideOutMax=[]  IntegratorContinuousStateAttributes=''  IntegratorStateMustResolveToSignalObject=off  IntegratorRTWStateStorageClass=Auto  FilterContinuousStateAttributes=''  FilterStateMustResolveToSignalObject=off  FilterRTWStateStorageClass=Auto  ParallelPVariant=InternalParameters  IdealPVariant=Disabled  IVariant=Disabled  DVariant=Disabled  IntegratorVariant=Disabled  SatVariant=Disabled  AWVariant=Disabled  PCopyVariant=Disabled  TRVariant=Disabled  FdbkBlocksVariant=Forward  IdealPFdbkVariant=Disabled  SatFdbkVariant=Disabled  DerivativeFilterVariant=Disabled  NVariant=Disabled  NCopyVariant=Disabled_SignalSpec  FilterICVariant=Disabled  IntegratorICVariant=Disabled  ExternalResetVariant=Disabled  TRSumVariant=Passthrough  SumFdbkVariant=Disabled  SumVariant=Passthrough_P
  C_vel_Z : simulink/Continuous/PID Controller  Controller=P  Form=Parallel  TimeDomain=Discrete-time  SampleTime=ctrl_Ts  IntegratorMethod=Forward Euler  FilterMethod=Forward Euler  ControllerParametersSource=internal  P=ctrl_Kp_v_pos  I=ctrl_Ki_vel  D=0  UseFilter=on  N=100  TunerSelectOption=Transfer Function Based (PID Tuner App)  InitialConditionSource=internal  InitialConditionForIntegrator=0  InitialConditionForFilter=0  DifferentiatorICPrevScaledInput=0  ExternalReset=rising  TrackingMode=off  Kt=1  LimitOutput=off  UpperSaturationLimit=inf  LowerSaturationLimit=-inf  LinearizeAsGain=on  AntiWindupMode=none  Kb=1  POutMin=[]  POutMax=[]  IOutMin=[]  IOutMax=[]  DOutMin=[]  DOutMax=[]  NOutMin=[]  NOutMax=[]  SumOutMin=[]  SumOutMax=[]  SaturationOutMin=[]  SaturationOutMax=[]  PParamMin=[]  PParamMax=[]  IParamMin=[]  IParamMax=[]  DParamMin=[]  DParamMax=[]  NParamMin=[]  NParamMax=[]  KbParamMin=[]  KbParamMax=[]  KtParamMin=[]  KtParamMax=[]  KbOutMin=[]  KbOutMax=[]  KtOutMin=[]  KtOutMax=[]  IntegratorOutMin=[]  IntegratorOutMax=[]  FilterOutMin=[]  FilterOutMax=[]  SumI1OutMin=[]  SumI1OutMax=[]  SumI2OutMin=[]  SumI2OutMax=[]  SumI3OutMin=[]  SumI3OutMax=[]  SumI4OutMin=[]  SumI4OutMax=[]  SumDOutMin=[]  SumDOutMax=[]  DifferentiatorOutMin=[]  DifferentiatorOutMax=[]  FilterDiffOutCoefMin=[]  FilterDiffOutCoefMax=[]  ReciprocalOutMin=[]  ReciprocalOutMax=[]  SumDenOutMin=[]  SumDenOutMax=[]  SumNumOutMin=[]  SumNumOutMax=[]  DivideOutMin=[]  DivideOutMax=[]  IntegratorContinuousStateAttributes=''  IntegratorStateMustResolveToSignalObject=off  IntegratorRTWStateStorageClass=Auto  FilterContinuousStateAttributes=''  FilterStateMustResolveToSignalObject=off  FilterRTWStateStorageClass=Auto  ParallelPVariant=InternalParameters  IdealPVariant=Disabled  IVariant=Disabled  DVariant=Disabled  IntegratorVariant=Disabled  SatVariant=Disabled  AWVariant=Disabled  PCopyVariant=Disabled  TRVariant=Disabled  FdbkBlocksVariant=Forward  IdealPFdbkVariant=Disabled  SatFdbkVariant=Disabled  DerivativeFilterVariant=Disabled  NVariant=Disabled  NCopyVariant=Disabled_SignalSpec  FilterICVariant=Disabled  IntegratorICVariant=Disabled  ExternalResetVariant=Disabled  TRSumVariant=Passthrough  SumFdbkVariant=Disabled  SumVariant=Passthrough_P
  Constant : Constant  Value=0
  Constant1 : Constant  Value=0
  Demux : Demux  Outputs=3
  Demux1 : Demux  Outputs=3
  Gain : Constant  Value=ctrl_k_pos
  Mux : Mux  Inputs=6
  Sum1 : Sum  Inputs=+|+|-
  Sum2 : Sum  Inputs=+|+|-
  Sum3 : Sum  Inputs=++|
  Sum4 : Sum  Inputs=++-
  Sum6 : Sum  Inputs=|++
  Sum7 : Sum  Inputs=++|
  Switch : Switch  Criteria=u2 ~= 0  Threshold=0.5
  Switch1 : Switch  Criteria=u2 ~= 0  Threshold=0.5
  abs_integrator1 : Subsystem
  abs_integrator2 : Subsystem
  tau_ang : Constant  Value=0
  tau_pos : Outport  VectorParamsAs1DForOutWhenUnconnected=off
  wires:
  Demux/1 -> C_pos_X/1(pos)
  Sum1/1 -> abs_integrator2/1(err_vx), C_vel_X/1
  Sum2/1 -> C_vel_Y/1, abs_integrator2/2(err_vy)
  Demux/2 -> C_pos_Y/1(pos)
  Demux1/1 -> Sum1/3
  Demux1/3 -> Sum4/3
  vel/1 -> Demux1/1
  Sum6/1 -> Mux/1
  Sum7/1 -> Mux/2
  Sum3/1 -> Mux/3
  tau_ang/1 -> Mux/6, Mux/5, Mux/4
  Gain/1 -> C_pos_Z/2(k), C_pos_Y/2(k), C_pos_X/2(k)
  enable/1 -> Switch/2, abs_integrator2/4(enabler), abs_integrator1/4(enabler), Switch1/2
  Mux/1 -> Switch/1
  Switch/1 -> tau_pos/1
  Constant/1 -> Switch/3
  Constant1/1 -> Switch1/3
  Switch1/1 -> Demux/1
  Sum4/1 -> abs_integrator2/3(err_vz), C_vel_Z/1
  err_pos/1 -> Switch1/1
  Demux/3 -> C_pos_Z/1(pos)
  C_pos_Z/2(vel) -> Sum4/2
  Demux1/2 -> Sum2/3
  C_pos_Y/2(vel) -> Sum2/2
  C_pos_X/1(err_int) -> abs_integrator1/1(err_x)
  C_pos_Z/1(err_int) -> abs_integrator1/3(err_z)
  C_pos_Y/1(err_int) -> abs_integrator1/2(err_y)
  C_pos_X/2(vel) -> Sum1/1
  abs_integrator1/3(int_z) -> Sum4/1
  abs_integrator1/2(int_y) -> Sum2/1
  abs_integrator1/1(int_x) -> Sum1/2
  C_vel_Y/1 -> Sum7/2
  C_vel_Z/1 -> Sum3/2
  abs_integrator2/1(int_vx) -> Sum6/2
  C_vel_X/1 -> Sum6/1
  abs_integrator2/2(int_vy) -> Sum7/1
  abs_integrator2/3(int_vz) -> Sum3/1

== system sim_all_2019b/Controller_mk4_v3/C_vel ==
  note: CONSIDERAZIONI:
      | - il controllore è un PI costruito con sisotool
      | - il modello considerato è su un singolo asse con massa e damping
  err_vel : Inport
  enable : Inport  Port=2
  C_vel_X : simulink/Continuous/PID Controller  Controller=P  Form=Parallel  TimeDomain=Discrete-time  SampleTime=ctrl_Ts  IntegratorMethod=Forward Euler  FilterMethod=Forward Euler  ControllerParametersSource=internal  P=ctrl_Kp_vel  I=ctrl_Ki_vel  D=0  UseFilter=on  N=100  TunerSelectOption=Transfer Function Based (PID Tuner App)  InitialConditionSource=internal  InitialConditionForIntegrator=0  InitialConditionForFilter=0  DifferentiatorICPrevScaledInput=0  ExternalReset=rising  TrackingMode=off  Kt=1  LimitOutput=off  UpperSaturationLimit=inf  LowerSaturationLimit=-inf  LinearizeAsGain=on  AntiWindupMode=none  Kb=1  POutMin=[]  POutMax=[]  IOutMin=[]  IOutMax=[]  DOutMin=[]  DOutMax=[]  NOutMin=[]  NOutMax=[]  SumOutMin=[]  SumOutMax=[]  SaturationOutMin=[]  SaturationOutMax=[]  PParamMin=[]  PParamMax=[]  IParamMin=[]  IParamMax=[]  DParamMin=[]  DParamMax=[]  NParamMin=[]  NParamMax=[]  KbParamMin=[]  KbParamMax=[]  KtParamMin=[]  KtParamMax=[]  KbOutMin=[]  KbOutMax=[]  KtOutMin=[]  KtOutMax=[]  IntegratorOutMin=[]  IntegratorOutMax=[]  FilterOutMin=[]  FilterOutMax=[]  SumI1OutMin=[]  SumI1OutMax=[]  SumI2OutMin=[]  SumI2OutMax=[]  SumI3OutMin=[]  SumI3OutMax=[]  SumI4OutMin=[]  SumI4OutMax=[]  SumDOutMin=[]  SumDOutMax=[]  DifferentiatorOutMin=[]  DifferentiatorOutMax=[]  FilterDiffOutCoefMin=[]  FilterDiffOutCoefMax=[]  ReciprocalOutMin=[]  ReciprocalOutMax=[]  SumDenOutMin=[]  SumDenOutMax=[]  SumNumOutMin=[]  SumNumOutMax=[]  DivideOutMin=[]  DivideOutMax=[]  IntegratorContinuousStateAttributes=''  IntegratorStateMustResolveToSignalObject=off  IntegratorRTWStateStorageClass=Auto  FilterContinuousStateAttributes=''  FilterStateMustResolveToSignalObject=off  FilterRTWStateStorageClass=Auto  ParallelPVariant=InternalParameters  IdealPVariant=Disabled  IVariant=Disabled  DVariant=Disabled  IntegratorVariant=Disabled  SatVariant=Disabled  AWVariant=Disabled  PCopyVariant=Disabled  TRVariant=Disabled  FdbkBlocksVariant=Forward  IdealPFdbkVariant=Disabled  SatFdbkVariant=Disabled  DerivativeFilterVariant=Disabled  NVariant=Disabled  NCopyVariant=Disabled_SignalSpec  FilterICVariant=Disabled  IntegratorICVariant=Disabled  ExternalResetVariant=Disabled  TRSumVariant=Passthrough  SumFdbkVariant=Disabled  SumVariant=Passthrough_P
  C_vel_Y : simulink/Continuous/PID Controller  Controller=P  Form=Parallel  TimeDomain=Discrete-time  SampleTime=ctrl_Ts  IntegratorMethod=Forward Euler  FilterMethod=Forward Euler  ControllerParametersSource=internal  P=ctrl_Kp_vel  I=ctrl_Ki_vel  D=0  UseFilter=on  N=100  TunerSelectOption=Transfer Function Based (PID Tuner App)  InitialConditionSource=internal  InitialConditionForIntegrator=0  InitialConditionForFilter=0  DifferentiatorICPrevScaledInput=0  ExternalReset=rising  TrackingMode=off  Kt=1  LimitOutput=off  UpperSaturationLimit=inf  LowerSaturationLimit=-inf  LinearizeAsGain=on  AntiWindupMode=none  Kb=1  POutMin=[]  POutMax=[]  IOutMin=[]  IOutMax=[]  DOutMin=[]  DOutMax=[]  NOutMin=[]  NOutMax=[]  SumOutMin=[]  SumOutMax=[]  SaturationOutMin=[]  SaturationOutMax=[]  PParamMin=[]  PParamMax=[]  IParamMin=[]  IParamMax=[]  DParamMin=[]  DParamMax=[]  NParamMin=[]  NParamMax=[]  KbParamMin=[]  KbParamMax=[]  KtParamMin=[]  KtParamMax=[]  KbOutMin=[]  KbOutMax=[]  KtOutMin=[]  KtOutMax=[]  IntegratorOutMin=[]  IntegratorOutMax=[]  FilterOutMin=[]  FilterOutMax=[]  SumI1OutMin=[]  SumI1OutMax=[]  SumI2OutMin=[]  SumI2OutMax=[]  SumI3OutMin=[]  SumI3OutMax=[]  SumI4OutMin=[]  SumI4OutMax=[]  SumDOutMin=[]  SumDOutMax=[]  DifferentiatorOutMin=[]  DifferentiatorOutMax=[]  FilterDiffOutCoefMin=[]  FilterDiffOutCoefMax=[]  ReciprocalOutMin=[]  ReciprocalOutMax=[]  SumDenOutMin=[]  SumDenOutMax=[]  SumNumOutMin=[]  SumNumOutMax=[]  DivideOutMin=[]  DivideOutMax=[]  IntegratorContinuousStateAttributes=''  IntegratorStateMustResolveToSignalObject=off  IntegratorRTWStateStorageClass=Auto  FilterContinuousStateAttributes=''  FilterStateMustResolveToSignalObject=off  FilterRTWStateStorageClass=Auto  ParallelPVariant=InternalParameters  IdealPVariant=Disabled  IVariant=Disabled  DVariant=Disabled  IntegratorVariant=Disabled  SatVariant=Disabled  AWVariant=Disabled  PCopyVariant=Disabled  TRVariant=Disabled  FdbkBlocksVariant=Forward  IdealPFdbkVariant=Disabled  SatFdbkVariant=Disabled  DerivativeFilterVariant=Disabled  NVariant=Disabled  NCopyVariant=Disabled_SignalSpec  FilterICVariant=Disabled  IntegratorICVariant=Disabled  ExternalResetVariant=Disabled  TRSumVariant=Passthrough  SumFdbkVariant=Disabled  SumVariant=Passthrough_P
  C_vel_Z : simulink/Continuous/PID Controller  Controller=P  Form=Parallel  TimeDomain=Discrete-time  SampleTime=ctrl_Ts  IntegratorMethod=Forward Euler  FilterMethod=Forward Euler  ControllerParametersSource=internal  P=ctrl_Kp_vel  I=ctrl_Ki_vel  D=0  UseFilter=on  N=100  TunerSelectOption=Transfer Function Based (PID Tuner App)  InitialConditionSource=internal  InitialConditionForIntegrator=0  InitialConditionForFilter=0  DifferentiatorICPrevScaledInput=0  ExternalReset=rising  TrackingMode=off  Kt=1  LimitOutput=off  UpperSaturationLimit=inf  LowerSaturationLimit=-inf  LinearizeAsGain=on  AntiWindupMode=none  Kb=1  POutMin=[]  POutMax=[]  IOutMin=[]  IOutMax=[]  DOutMin=[]  DOutMax=[]  NOutMin=[]  NOutMax=[]  SumOutMin=[]  SumOutMax=[]  SaturationOutMin=[]  SaturationOutMax=[]  PParamMin=[]  PParamMax=[]  IParamMin=[]  IParamMax=[]  DParamMin=[]  DParamMax=[]  NParamMin=[]  NParamMax=[]  KbParamMin=[]  KbParamMax=[]  KtParamMin=[]  KtParamMax=[]  KbOutMin=[]  KbOutMax=[]  KtOutMin=[]  KtOutMax=[]  IntegratorOutMin=[]  IntegratorOutMax=[]  FilterOutMin=[]  FilterOutMax=[]  SumI1OutMin=[]  SumI1OutMax=[]  SumI2OutMin=[]  SumI2OutMax=[]  SumI3OutMin=[]  SumI3OutMax=[]  SumI4OutMin=[]  SumI4OutMax=[]  SumDOutMin=[]  SumDOutMax=[]  DifferentiatorOutMin=[]  DifferentiatorOutMax=[]  FilterDiffOutCoefMin=[]  FilterDiffOutCoefMax=[]  ReciprocalOutMin=[]  ReciprocalOutMax=[]  SumDenOutMin=[]  SumDenOutMax=[]  SumNumOutMin=[]  SumNumOutMax=[]  DivideOutMin=[]  DivideOutMax=[]  IntegratorContinuousStateAttributes=''  IntegratorStateMustResolveToSignalObject=off  IntegratorRTWStateStorageClass=Auto  FilterContinuousStateAttributes=''  FilterStateMustResolveToSignalObject=off  FilterRTWStateStorageClass=Auto  ParallelPVariant=InternalParameters  IdealPVariant=Disabled  IVariant=Disabled  DVariant=Disabled  IntegratorVariant=Disabled  SatVariant=Disabled  AWVariant=Disabled  PCopyVariant=Disabled  TRVariant=Disabled  FdbkBlocksVariant=Forward  IdealPFdbkVariant=Disabled  SatFdbkVariant=Disabled  DerivativeFilterVariant=Disabled  NVariant=Disabled  NCopyVariant=Disabled_SignalSpec  FilterICVariant=Disabled  IntegratorICVariant=Disabled  ExternalResetVariant=Disabled  TRSumVariant=Passthrough  SumFdbkVariant=Disabled  SumVariant=Passthrough_P
  Constant3 : Constant  Value=0
  Constant4 : Constant  Value=0
  Constant5 : Constant  Value=0
  Demux1 : Demux  Outputs=3
  Mux2 : Mux  Inputs=6
  Sum5 : Sum  Inputs=++|
  Sum7 : Sum  Inputs=|++
  Sum8 : Sum  Inputs=++|
  Switch2 : Switch  Criteria=u2 ~= 0  Threshold=0.5
  Switch3 : Switch  Criteria=u2 ~= 0  Threshold=0.5
  abs_integrator : Subsystem
  tau_vel1 : Outport  VectorParamsAs1DForOutWhenUnconnected=off
  wires:
  C_vel_Y/1 -> Sum8/2
  C_vel_X/1 -> Sum7/1
  abs_integrator/1(int_vx) -> Sum7/2
  abs_integrator/3(int_vz) -> Sum5/1
  C_vel_Z/1 -> Sum5/2
  abs_integrator/2(int_vy) -> Sum8/1
  Switch2/1 -> Demux1/1
  err_vel/1 -> Switch2/1
  Constant3/1 -> Switch2/3
  Demux1/2 -> abs_integrator/2(err_vy), C_vel_Y/1
  Demux1/1 -> abs_integrator/1(err_vx), C_vel_X/1
  Demux1/3 -> C_vel_Z/1, abs_integrator/3(err_vz)
  Switch3/1 -> tau_vel1/1
  Mux2/1 -> Switch3/1
  Sum7/1 -> Mux2/1
  enable/1 -> abs_integrator/4(enabler), Switch3/2, Switch2/2
  Constant5/1 -> Switch3/3
  Sum5/1 -> Mux2/3
  Sum8/1 -> Mux2/2
  Constant4/1 -> Mux2/6, Mux2/5, Mux2/4

== system sim_all_2019b/Controller_mk4_v3/InputOr_Organizer ==
  prof_trig : Inport
  or_d : Inport  Port=2
  or_s : Inport  Port=3
  orp_ned : Inport  Port=4
  Switch4 : Switch  Criteria=u2 > Threshold  Threshold=0.5
  diff_or : MATLAB Function  TreatAsAtomicUnit=on
  err_or : Outport
  wires:
  diff_or/1(err_or) -> err_or/1
  Switch4/1 -> diff_or/1(or_d)
  prof_trig/1 -> Switch4/2
  or_d/1 -> Switch4/1
  orp_ned/1 -> Switch4/3
  or_s/1 -> diff_or/2(or_s)

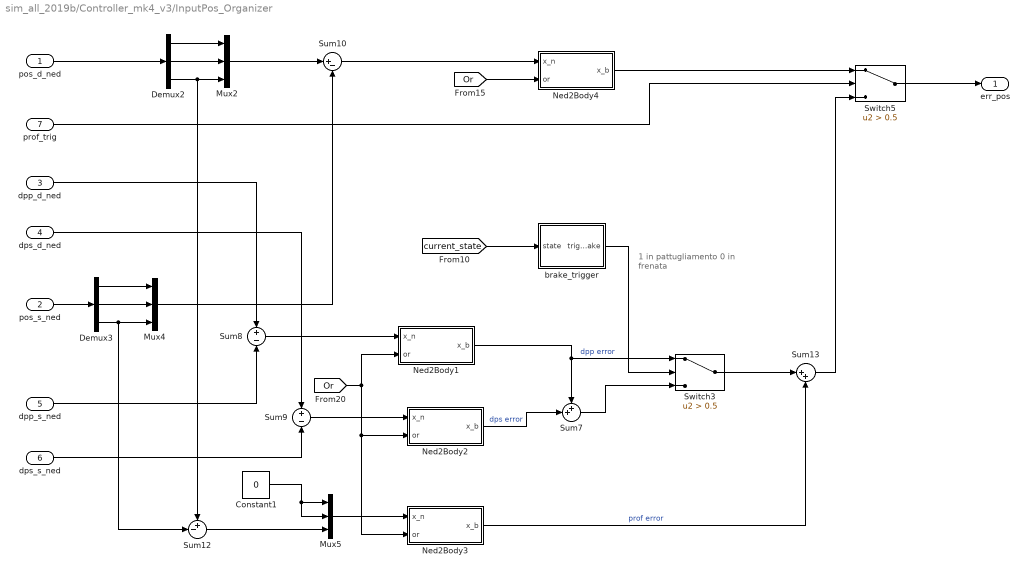
== system sim_all_2019b/Controller_mk4_v3/InputPos_Organizer ==
  note: 1 in pattugliamento
      | 0 in frenata
  pos_d_ned : Inport
  pos_s_ned : Inport  Port=2
  dpp_d_ned : Inport  Port=3
  dps_d_ned : Inport  Port=4
  dpp_s_ned : Inport  Port=5
  dps_s_ned : Inport  Port=6
  prof_trig : Inport  Port=7
  Constant1 : Constant  Value=0
  Demux2 : Demux  Outputs=3
  Demux3 : Demux  Outputs=3
  Mux2 : Mux  Inputs=3
  Mux4 : Mux  Inputs=3
  Mux5 : Mux  Inputs=3
  Ned2Body1 : MATLAB Function  TreatAsAtomicUnit=on
  Ned2Body2 : MATLAB Function  TreatAsAtomicUnit=on
  Ned2Body3 : MATLAB Function  TreatAsAtomicUnit=on
  Ned2Body4 : MATLAB Function  TreatAsAtomicUnit=on
  Sum10 : Sum  Inputs=|+-
  Sum12 : Sum  Inputs=+-|
  Sum13 : Sum  Inputs=|++
  Sum7 : Sum  Inputs=++|
  Sum8 : Sum  Inputs=+|-
  Sum9 : Sum  Inputs=+|-
  Switch3 : Switch  Criteria=u2 > Threshold  Threshold=0.5
  Switch5 : Switch  Criteria=u2 > Threshold  Threshold=0.5
  brake_trigger : MATLAB Function  TreatAsAtomicUnit=on
  err_pos : Outport
  wires:
  Sum13/1 -> Switch5/3
  Sum10/1 -> Ned2Body4/1(x_n)
  brake_trigger/1(trigg_brake) -> Switch3/2
  [Or] -> Ned2Body1/2(or), Ned2Body3/2(or), Ned2Body2/2(or)
  Switch3/1 -> Sum13/1
  Mux2/1 -> Sum10/1
  Switch5/1 -> err_pos/1
  Mux5/1 -> Ned2Body3/1(x_n)
  prof_trig/1 -> Switch5/2
  Ned2Body2/1(x_b) -> Sum7/2  "dps error"
  Ned2Body3/1(x_b) -> Sum13/2  "prof error"
  Sum8/1 -> Ned2Body1/1(x_n)
  dpp_d_ned/1 -> Sum8/1
  Demux2/3 -> Mux2/3, Sum12/1
  Mux4/1 -> Sum10/2
  Demux2/2 -> Mux2/2
  Ned2Body4/1(x_b) -> Switch5/1
  [Or] -> Ned2Body4/2(or)
  Demux3/3 -> Mux4/3, Sum12/2
  Ned2Body1/1(x_b) -> Switch3/1, Sum7/1  "dpp error"
  Demux2/1 -> Mux2/1
  Sum12/1 -> Mux5/3
  [current_state] -> brake_trigger/1(state)
  Sum9/1 -> Ned2Body2/1(x_n)
  Demux3/2 -> Mux4/2
  Constant1/1 -> Mux5/2, Mux5/1
  Sum7/1 -> Switch3/3
  Demux3/1 -> Mux4/1
  pos_s_ned/1 -> Demux3/1
  dps_s_ned/1 -> Sum9/2
  pos_d_ned/1 -> Demux2/1
  dps_d_ned/1 -> Sum9/1
  dpp_s_ned/1 -> Sum8/2

== system sim_all_2019b/Controller_mk4_v3/InputVel_Organizer ==
  vel_d_ned : Inport
  vel_s_body : Inport  Port=2
  Ned2Body4 : MATLAB Function  TreatAsAtomicUnit=on
  Sum11 : Sum  Inputs=|+-
  err_vel : Outport
  wires:
  Ned2Body4/1(x_b) -> Sum11/1
  vel_d_ned/1 -> Ned2Body4/1(x_n)
  Sum11/1 -> err_vel/1
  vel_s_body/1 -> Sum11/2
  [Or] -> Ned2Body4/2(or)

== system sim_all_2019b/Controller_mk4_v3/Mixer ==
  tau_pos : Inport
  tau_vel : Inport  Port=2
  tau_or : Inport  Port=3
  Mix : MATLAB Function  TreatAsAtomicUnit=on  SystemSampleTime=ctrl_Ts
  T2n : MATLAB Function  TreatAsAtomicUnit=on  SystemSampleTime=ctrl_Ts
  TAM1 : cstblocks/LTI System  sys=inv(ctrl_TAM)  IC=[]
  TAM2 : cstblocks/LTI System  sys=inv(ctrl_TAM)  IC=[]
  TAM3 : cstblocks/LTI System  sys=inv(ctrl_TAM)  IC=[]
  n : Outport  VectorParamsAs1DForOutWhenUnconnected=off
  wires:
  Mix/1(T) -> T2n/1(T)
  TAM3/1 -> Mix/3(To)
  TAM2/1 -> Mix/2(Tv)
  TAM1/1 -> Mix/1(Tp)
  tau_pos/1 -> TAM1/1
  tau_vel/1 -> TAM2/1
  T2n/1(n) -> n/1
  tau_or/1 -> TAM3/1

== system sim_all_2019b/Controller_mk4_v3/signal_to_NED ==
  Vel_d : Inport
  Dpp_d : Inport  Port=2
  Dps_d : Inport  Port=3
  Orp_d : Inport  Port=4
  Dpp_s : Inport  Port=5
  Dps_s : Inport  Port=6
  Signal_d->NED : Subsystem
  Signal_s->NED : Subsystem
  prof_trigger : MATLAB Function  TreatAsAtomicUnit=on
  Dpp_d_ned : Outport
  Dps_d_ned : Outport  Port=2
  Dpp_s_ned : Outport  Port=3
  Dps_s_ned : Outport  Port=4
  trigg_prof : Outport  Port=5
  Vel_d_ned : Outport  Port=6
  Orp_d_ned : Outport  Port=7
  wires:
  Dps_s/1 -> Signal_s->NED/2(Dps_s)
  [current_state] -> prof_trigger/1(state)
  [parete_attuale] -> Signal_d->NED/5(Wall)
  [parete_attuale] -> Signal_s->NED/3(Wall)
  Signal_d->NED/4(Orp_d_ned) -> Orp_d_ned/1
  Vel_d/1 -> Signal_d->NED/1(Vel_d)
  Dpp_d/1 -> Signal_d->NED/2(Dpp_d)
  Signal_d->NED/3(Dps_d_ned) -> Dps_d_ned/1
  Signal_d->NED/2(Dpp_d_ned) -> Dpp_d_ned/1
  Orp_d/1 -> Signal_d->NED/4(Orp_d)
  Dps_d/1 -> Signal_d->NED/3(Dps_d)
  Signal_s->NED/2(Dps_s_ned) -> Dps_s_ned/1
  Dpp_s/1 -> Signal_s->NED/1(Dpp_s)
  prof_trigger/1(trigg_prof) -> trigg_prof/1
  Signal_s->NED/1(Dpp_s_ned) -> Dpp_s_ned/1
  Signal_d->NED/1(Vel_d_ned) -> Vel_d_ned/1
